simulink model "model_p7"  (R2020b)
settings: Solver=VariableStepAuto  StartTime=0.0  StopTime=10.0  RelTol=1e-3
settings Model: Creator=ADMIN  LastModifiedBy=ADMIN

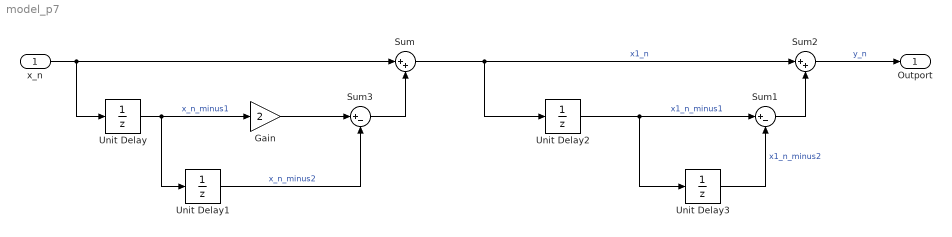
== system model_p7 ==
  x_n : Inport
  Gain : Gain  Gain=2
  Sum : Sum  Inputs=|++
  Sum1 : Sum  Inputs=|+-
  Sum2 : Sum  Inputs=|++
  Sum3 : Sum  Inputs=|+-
  Unit Delay{,1..3} (4 alike) : UnitDelay  SampleTime=-1  HasFrameUpgradeWarning=on
  Outport : Outport
  wires:
  x_n/1 -> Unit Delay/1, Sum/1
  Unit Delay/1 -> Unit Delay1/1, Gain/1  "x_n_minus1"
  Unit Delay1/1 -> Sum3/2  "x_n_minus2"
  Gain/1 -> Sum3/1
  Sum3/1 -> Sum/2
  Sum/1 -> Unit Delay2/1, Sum2/1  "x1_n"
  Unit Delay2/1 -> Unit Delay3/1, Sum1/1  "x1_n_minus1"
  Sum1/1 -> Sum2/2
  Unit Delay3/1 -> Sum1/2  "x1_n_minus2"
  Sum2/1 -> Outport/1  "y_n"
